simulink model "ES249A_MotAgCorrln"  (R2013b)
settings: Solver=FixedStepDiscrete  SolverMode=SingleTasking  StartTime=0.0  StopTime=1  FixedStep=0.002  RelTol=1e-3
undefined symbols (not defined in the file): FLTINJ_MOTAGCORRLN_MOTAGIDPTSIG, HALFREV_MOTREV_U0P16, MOTAGACORRLNST_CNT_U08, MotAgAMotAgBCorrln, MotAgAMotAgCCorrln, MOTAGBCORRLNST_CNT_U08, MotAgBMotAgCCorrln, MOTAGCCORRLNST_CNT_U08, MOTAGCORRLNERRTHD_MOTREVELEC_U0P16, MOTAGCORRLNNTCFAILSTEP_CNT_U16, MOTAGCORRLNNTCPASSSTEP_CNT_U16, MOTAGMAXSTALLCNTR_CNT_U08, MotAgMeclCorrlnSt, MotAgMeclIdptSig, NtcSts1, sigbuilder_block, SysGlbPrmMotPoleCnt
libraries: simulink x5
(part 3 of 4)

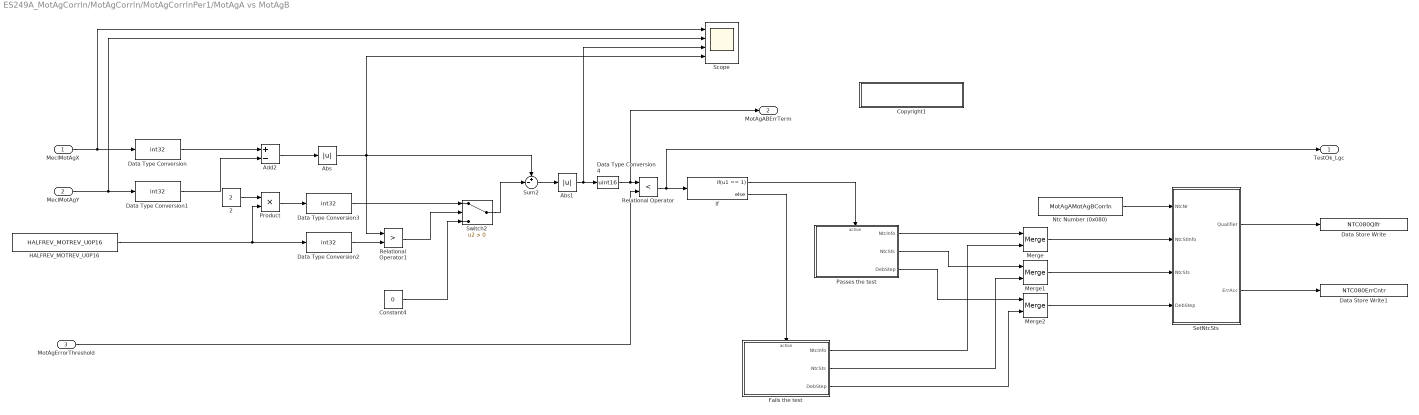
== system ES249A_MotAgCorrln/MotAgCorrln/MotAgCorrlnPer1/MotAgA vs MotAgB ==
  MeclMotAgX : Inport  RequirementInfo={} %GIDa_209a8ec2_f83a_4596_ac14_016e97e43532
  MeclMotAgY : Inport  RequirementInfo={} %GIDa_3879b633_065b_44db_a611_7209c5040c41  Port=2
  MotAgErrorThreshold : Inport  RequirementInfo={} %GIDa_52fd4367_99f4_419f_a569_0cba8f97a327  Port=3
  2 : Constant  Value=2  OutDataTypeStr=int32
  Abs : Abs
  Abs1 : Abs
  Add2 : Sum  Inputs=+-  AccumDataTypeStr=int32
  Constant4 : Constant  Value=0  OutDataTypeStr=int32
  Copyright1 : Subsystem  Description=|  RequirementInfo={} %GIDa_43863c04_fa5e_452c_a1b7_4fa30e8bd61b  mask(Copyright Information){none=on}
      | Copyright info block.                                               
      |                                                                     
      | Place copyright information at the top of every subsystem in design.
      mask prompts: none "No parameters"
      mask help: Place copyright information at the top of every subsystem in design.
      mask Display:
      | NxtrConf = 'Nexteer Confidential';
      | 
      | sys = bdroot; %handle for the current model ("system")
      | first = get_param(sys,'Created');
      | if(isempty(first))
      |     first = datestr(now,'yyyy');
      | else
      |     first = first(end-3:end);  %year is last four digits
      | end
      | 
      | last = get_param(sys,'LastModifiedDate');
      | if isempty(last)
      |     last = datestr(now,'yyyy');
      | else
      |     last = last(end-3:end);
      | end
      | 
      | if strcmp(first,last)
      |     fprintf('%s\nCopyright  %s Nexteer',NxtrConf,first);
      | else
      |     fprintf('%s\n%s%s-%s Nexteer',NxtrConf,char(169),first,last);
      | end
  Data Store Write : DataStoreWrite  RequirementInfo={} %GIDa_9512697d_c087_4109_9134_0a84db0896e8  DataStoreName=NTC080Qlfr
  Data Store Write1 : DataStoreWrite  RequirementInfo={} %GIDa_09fa0ad2_fadc_4e01_82b6_87880c397f4c  DataStoreName=NTC080ErrCntr
  Data Type Conversion{,1..3} (4 alike) : DataTypeConversion  OutDataTypeStr=int32
  Data Type Conversion4 : DataTypeConversion  OutDataTypeStr=uint16
  Fails the test : Subsystem  RequirementInfo={} %GIDa_32330a11_135a_4d4a_b6a9_5738b4884140  TreatAsAtomicUnit=on
  HALFREV_MOTREV_U0P16 : Constant  Value=HALFREV_MOTREV_U0P16  OutDataTypeStr=int32
  If : If  RequirementInfo={} %GIDa_4a7e1530_6c57_410a_8590_40bd88f14402  IfExpression=u1 == 1
  Merge : Merge  RequirementInfo={} %GIDa_5c5d4849_b0d7_417e_8e37_be493b9884db
  Merge1 : Merge  RequirementInfo={} %GIDa_96dc7a19_089f_4a81_91dd_98b954b09d33
  Merge2 : Merge  RequirementInfo={} %GIDa_445cf7d9_fe34_4f83_8f83_84d725eb67cd
  Ntc Number (0x080) : Constant  RequirementInfo={} %GIDa_17484570_857f_4649_8079_9998f179e352  Value=MotAgAMotAgBCorrln
  Passes the test : Subsystem  RequirementInfo={} %GIDa_2e2aa5eb_d2a7_4382_b0d6_a86d4a99b386  TreatAsAtomicUnit=on
  Product : Product
  Relational Operator : RelationalOperator  RequirementInfo={} %GIDa_e81e555f_20f9_4e1d_8333_9ac819d3840d  Operator=<  OutDataTypeStr=boolean
  Relational Operator1 : RelationalOperator  Operator=>  OutDataTypeStr=boolean
  Scope : Scope  NumInputPorts=4
      settings: TimeRange=1  YMin=0~-5~-5~-5  YMax=8~5~5~5
  SetNtcSts : Subsystem  RequirementInfo={} %GIDa_372e5e5c_ac16_4961_ac82_62e12ce3987b  TreatAsAtomicUnit=on
      settings: RTWSystemCode=Inline
  Sum2 : Sum  Inputs=+-|
  Switch2 : Switch  Criteria=u2 > Threshold
  TestOk_Lgc : Outport  RequirementInfo={} %GIDa_58faf550_67b9_443b_9b7a_437f5011a6c4
  MotAgABErrTerm : Outport  RequirementInfo={'linktype_rmi_doors' '0000c47a (/E-STEER Core/SubSystem Specifications/Electrical Actuator/Control Module/FDD Module Requirements/EA4/ES249A_MotAgCorrln)' '#ES249A_116' 'true' 'REQ: ES249A_116' '' } %GIDa_f792b4e5_8164_43e5_9c8c_3a51a3d2addb  Port=2
  wires:
  Relational Operator/1 -> If/1, TestOk_Lgc/1
  If/1 -> Passes the test/Action
  If/2 -> Fails the test/Action
  Ntc Number (0x080)/1 -> SetNtcSts/1(NtcNr)
  Merge/1 -> SetNtcSts/2(NtcStInfo)
  Merge1/1 -> SetNtcSts/3(NtcSts)
  Merge2/1 -> SetNtcSts/4(DebStep)
  Passes the test/1(NtcInfo) -> Merge/1
  Fails the test/1(NtcInfo) -> Merge/2
  Passes the test/2(NtcSts) -> Merge1/1
  Fails the test/2(NtcSts) -> Merge1/2
  Fails the test/3(DebStep) -> Merge2/2
  Passes the test/3(DebStep) -> Merge2/1
  SetNtcSts/1(Qualifier) -> Data Store Write/1
  SetNtcSts/2(ErrAcc) -> Data Store Write1/1
  MotAgErrorThreshold/1 -> Relational Operator/2
  Data Type Conversion/1 -> Add2/1
  Sum2/1 -> Abs1/1
  Data Type Conversion1/1 -> Add2/2
  Switch2/1 -> Sum2/2
  Constant4/1 -> Switch2/3
  Relational Operator1/1 -> Switch2/2
  HALFREV_MOTREV_U0P16/1 -> Product/2, Data Type Conversion2/1
  Abs/1 -> Scope/4, Sum2/1, Relational Operator1/1
  Add2/1 -> Abs/1
  MeclMotAgX/1 -> Scope/1, Data Type Conversion/1
  MeclMotAgY/1 -> Scope/2, Data Type Conversion1/1
  Data Type Conversion2/1 -> Relational Operator1/2
  2/1 -> Product/1
  Product/1 -> Data Type Conversion3/1
  Data Type Conversion3/1 -> Switch2/1
  Abs1/1 -> Data Type Conversion4/1, Scope/3
  Data Type Conversion4/1 -> Relational Operator/1, MotAgABErrTerm/1

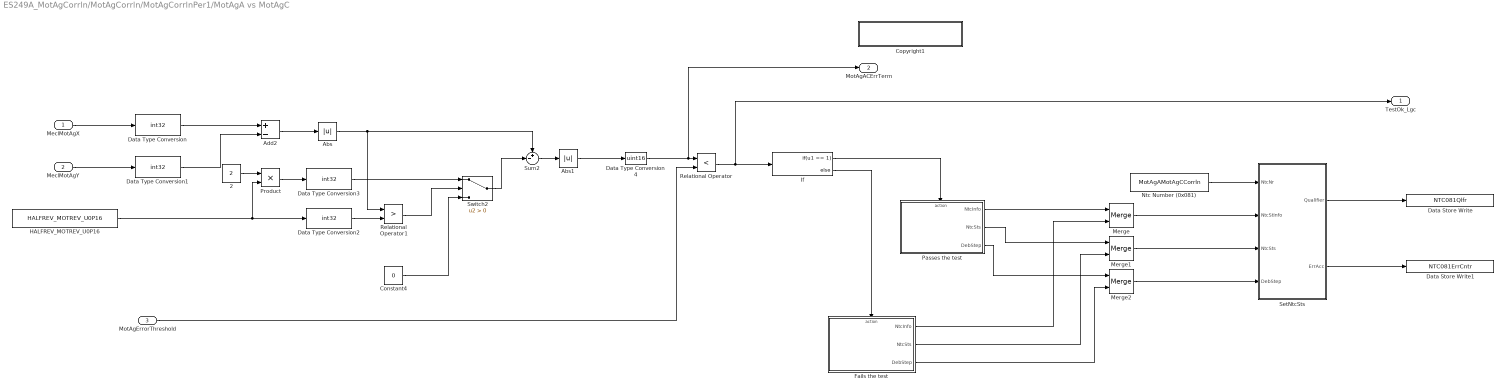
== system ES249A_MotAgCorrln/MotAgCorrln/MotAgCorrlnPer1/MotAgA vs MotAgC ==
  MeclMotAgX : Inport  RequirementInfo={} %GIDa_ca73f5b5_eafe_434b_a911_6609f3f516c8
  MeclMotAgY : Inport  RequirementInfo={} %GIDa_a43669f2_2345_43dd_8255_a23bf60027e6  Port=2
  MotAgErrorThreshold : Inport  RequirementInfo={} %GIDa_293d2f0c_7000_4fd4_9706_6d02dd117e93  Port=3
  2 : Constant  Value=2  OutDataTypeStr=int32
  Abs : Abs
  Abs1 : Abs
  Add2 : Sum  Inputs=+-  AccumDataTypeStr=int32
  Constant4 : Constant  Value=0  OutDataTypeStr=int32
  Copyright1 : Subsystem  Description=|  RequirementInfo={} %GIDa_2297f3bd_4d76_4488_9958_d579b77d02c1  mask(Copyright Information){none=on}
      | Copyright info block.                                               
      |                                                                     
      | Place copyright information at the top of every subsystem in design.
      mask prompts: none "No parameters"
      mask help: Place copyright information at the top of every subsystem in design.
      mask Display:
      | NxtrConf = 'Nexteer Confidential';
      | 
      | sys = bdroot; %handle for the current model ("system")
      | first = get_param(sys,'Created');
      | if(isempty(first))
      |     first = datestr(now,'yyyy');
      | else
      |     first = first(end-3:end);  %year is last four digits
      | end
      | 
      | last = get_param(sys,'LastModifiedDate');
      | if isempty(last)
      |     last = datestr(now,'yyyy');
      | else
      |     last = last(end-3:end);
      | end
      | 
      | if strcmp(first,last)
      |     fprintf('%s\nCopyright  %s Nexteer',NxtrConf,first);
      | else
      |     fprintf('%s\n%s%s-%s Nexteer',NxtrConf,char(169),first,last);
      | end
  Data Store Write : DataStoreWrite  RequirementInfo={} %GIDa_72478395_f981_454c_bb4d_0a88e45525f3  DataStoreName=NTC081Qlfr
  Data Store Write1 : DataStoreWrite  RequirementInfo={} %GIDa_0db287a0_3687_4b20_b932_4d814fe6d91c  DataStoreName=NTC081ErrCntr
  Data Type Conversion{,1..3} (4 alike) : DataTypeConversion  OutDataTypeStr=int32
  Data Type Conversion4 : DataTypeConversion  OutDataTypeStr=uint16
  Fails the test : Subsystem  RequirementInfo={} %GIDa_49fef5d6_5f11_4857_b273_ce522995cb73  TreatAsAtomicUnit=on
  HALFREV_MOTREV_U0P16 : Constant  Value=HALFREV_MOTREV_U0P16  OutDataTypeStr=int32
  If : If  RequirementInfo={} %GIDa_91b41173_b799_4940_951b_3ca3f1c91555  IfExpression=u1 == 1
  Merge : Merge  RequirementInfo={} %GIDa_14c5d993_a2fa_413b_a86d_168b64c7d573
  Merge1 : Merge  RequirementInfo={} %GIDa_c9320e0e_c294_4d17_8556_240a5cb0dfb1
  Merge2 : Merge  RequirementInfo={} %GIDa_945fcc23_377a_4219_9065_ef24679f88cd
  Ntc Number (0x081) : Constant  RequirementInfo={} %GIDa_e90d3b09_c43d_40da_938d_9d742c0ddf76  Value=MotAgAMotAgCCorrln
  Passes the test : Subsystem  RequirementInfo={} %GIDa_e126288c_26d5_4a45_ab77_0ce46127a866  TreatAsAtomicUnit=on
  Product : Product
  Relational Operator : RelationalOperator  RequirementInfo={} %GIDa_6ad4b311_7ce2_4d33_9521_311c03329a1b  Operator=<  OutDataTypeStr=boolean
  Relational Operator1 : RelationalOperator  Operator=>  OutDataTypeStr=boolean
  SetNtcSts : Subsystem  RequirementInfo={} %GIDa_7cf4e5eb_3813_4cd2_9ac5_e73cd08cc7f4  TreatAsAtomicUnit=on
      settings: RTWSystemCode=Inline
  Sum2 : Sum  Inputs=+-|
  Switch2 : Switch  Criteria=u2 > Threshold
  TestOk_Lgc : Outport  RequirementInfo={} %GIDa_0a018449_8aa2_4b67_9646_7371bac07a88
  MotAgACErrTerm : Outport  RequirementInfo={'linktype_rmi_doors' '0000c47a (/E-STEER Core/SubSystem Specifications/Electrical Actuator/Control Module/FDD Module Requirements/EA4/ES249A_MotAgCorrln)' '#ES249A_117' 'true' 'REQ: ES249A_117' '' } %GIDa_a2ba7b60_3fe2_4467_92e3_b3741369c184  Port=2
  wires:
  Relational Operator/1 -> If/1, TestOk_Lgc/1
  If/1 -> Passes the test/Action
  If/2 -> Fails the test/Action
  Ntc Number (0x081)/1 -> SetNtcSts/1(NtcNr)
  Merge/1 -> SetNtcSts/2(NtcStInfo)
  Merge1/1 -> SetNtcSts/3(NtcSts)
  Merge2/1 -> SetNtcSts/4(DebStep)
  Passes the test/1(NtcInfo) -> Merge/1
  Fails the test/1(NtcInfo) -> Merge/2
  Passes the test/2(NtcSts) -> Merge1/1
  Fails the test/2(NtcSts) -> Merge1/2
  Fails the test/3(DebStep) -> Merge2/2
  Passes the test/3(DebStep) -> Merge2/1
  SetNtcSts/1(Qualifier) -> Data Store Write/1
  SetNtcSts/2(ErrAcc) -> Data Store Write1/1
  Abs1/1 -> Data Type Conversion4/1
  MotAgErrorThreshold/1 -> Relational Operator/2
  Data Type Conversion/1 -> Add2/1
  Sum2/1 -> Abs1/1
  Data Type Conversion1/1 -> Add2/2
  Switch2/1 -> Sum2/2
  Constant4/1 -> Switch2/3
  Relational Operator1/1 -> Switch2/2
  HALFREV_MOTREV_U0P16/1 -> Product/2, Data Type Conversion2/1
  Abs/1 -> Sum2/1, Relational Operator1/1
  Add2/1 -> Abs/1
  MeclMotAgX/1 -> Data Type Conversion/1
  MeclMotAgY/1 -> Data Type Conversion1/1
  Data Type Conversion2/1 -> Relational Operator1/2
  2/1 -> Product/1
  Product/1 -> Data Type Conversion3/1
  Data Type Conversion3/1 -> Switch2/1
  Data Type Conversion4/1 -> MotAgACErrTerm/1, Relational Operator/1

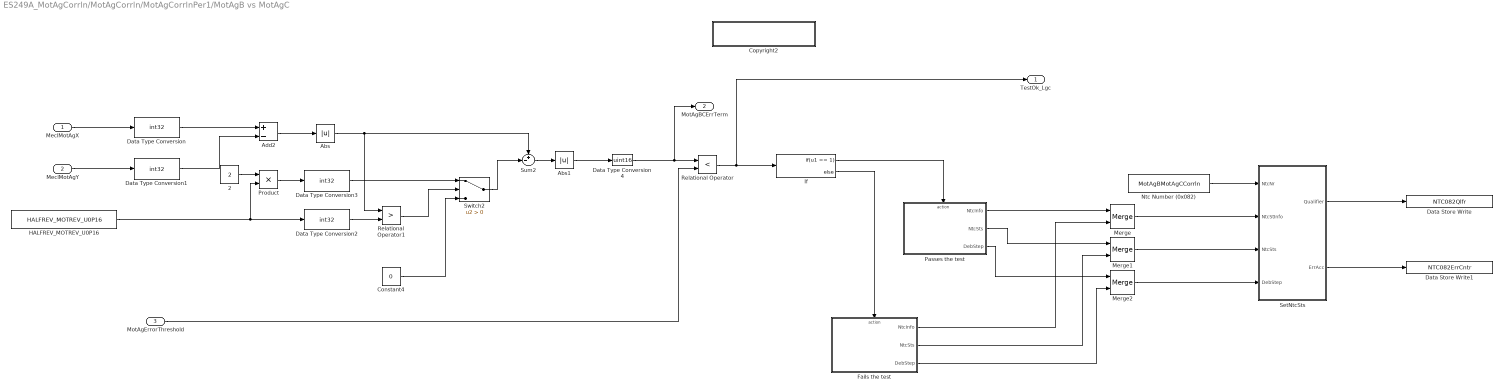
== system ES249A_MotAgCorrln/MotAgCorrln/MotAgCorrlnPer1/MotAgB vs MotAgC ==
  MeclMotAgX : Inport  RequirementInfo={} %GIDa_bf924aab_b5c7_4b3c_951d_c0fbe0c1bb55
  MeclMotAgY : Inport  RequirementInfo={} %GIDa_07ad9c05_b7c9_4d10_b318_38953ab658a8  Port=2
  MotAgErrorThreshold : Inport  RequirementInfo={} %GIDa_2cb4bb85_3f7a_48b7_a9d1_04f72aa7a276  Port=3
  2 : Constant  Value=2  OutDataTypeStr=int32
  Abs : Abs
  Abs1 : Abs
  Add2 : Sum  Inputs=+-  AccumDataTypeStr=int32
  Constant4 : Constant  Value=0  OutDataTypeStr=int32
  Copyright2 : Subsystem  Description=|  RequirementInfo={} %GIDa_151a706e_d981_4739_b788_73043061d7fb  mask(Copyright Information){none=on}
      | Copyright info block.                                               
      |                                                                     
      | Place copyright information at the top of every subsystem in design.
      mask prompts: none "No parameters"
      mask help: Place copyright information at the top of every subsystem in design.
      mask Display:
      | NxtrConf = 'Nexteer Confidential';
      | 
      | sys = bdroot; %handle for the current model ("system")
      | first = get_param(sys,'Created');
      | if(isempty(first))
      |     first = datestr(now,'yyyy');
      | else
      |     first = first(end-3:end);  %year is last four digits
      | end
      | 
      | last = get_param(sys,'LastModifiedDate');
      | if isempty(last)
      |     last = datestr(now,'yyyy');
      | else
      |     last = last(end-3:end);
      | end
      | 
      | if strcmp(first,last)
      |     fprintf('%s\nCopyright  %s Nexteer',NxtrConf,first);
      | else
      |     fprintf('%s\n%s%s-%s Nexteer',NxtrConf,char(169),first,last);
      | end
  Data Store Write : DataStoreWrite  RequirementInfo={} %GIDa_8eb81dab_454a_49f7_9b16_ac976242f325  DataStoreName=NTC082Qlfr
  Data Store Write1 : DataStoreWrite  RequirementInfo={} %GIDa_63ee642a_2bfa_48da_987e_40de90a1b8a9  DataStoreName=NTC082ErrCntr
  Data Type Conversion{,1..3} (4 alike) : DataTypeConversion  OutDataTypeStr=int32
  Data Type Conversion4 : DataTypeConversion  OutDataTypeStr=uint16
  "Fails the test " : Subsystem  RequirementInfo={} %GIDa_f8fb0c70_978f_4e3b_983d_e2d82756bf9b  TreatAsAtomicUnit=on
  HALFREV_MOTREV_U0P16 : Constant  Value=HALFREV_MOTREV_U0P16  OutDataTypeStr=int32
  If : If  RequirementInfo={} %GIDa_d8e22f8c_9e8f_4fa2_b4a1_01dc402be394  IfExpression=u1 == 1
  Merge : Merge  RequirementInfo={} %GIDa_6b0bb93a_8c69_4319_8a50_13213446c0d5
  Merge1 : Merge  RequirementInfo={} %GIDa_af68ae2f_d22d_4760_a231_9874859d41d2
  Merge2 : Merge  RequirementInfo={} %GIDa_e2802f96_b723_4964_a51f_af2ea2fa5b23
  Ntc Number (0x082) : Constant  RequirementInfo={} %GIDa_e1189385_ef24_4fb2_b048_68c7cb7489b1  Value=MotAgBMotAgCCorrln
  Passes the test : Subsystem  RequirementInfo={} %GIDa_82b55705_08f4_4798_b701_46f5356af831  TreatAsAtomicUnit=on
  Product : Product
  Relational Operator : RelationalOperator  RequirementInfo={} %GIDa_38fe0bde_8c6d_4ad7_8dea_b59dbfe668f4  Operator=<  OutDataTypeStr=boolean
  Relational Operator1 : RelationalOperator  Operator=>  OutDataTypeStr=boolean
  SetNtcSts : Subsystem  RequirementInfo={} %GIDa_647bea77_8184_4d0a_9df9_898d529ac2c2  TreatAsAtomicUnit=on
      settings: RTWSystemCode=Inline
  Sum2 : Sum  Inputs=+-|
  Switch2 : Switch  Criteria=u2 > Threshold
  TestOk_Lgc : Outport  RequirementInfo={} %GIDa_45ded846_667e_422a_9bd3_12a64f3f619d
  MotAgBCErrTerm : Outport  RequirementInfo={'linktype_rmi_doors' '0000c47a (/E-STEER Core/SubSystem Specifications/Electrical Actuator/Control Module/FDD Module Requirements/EA4/ES249A_MotAgCorrln)' '#ES249A_118' 'true' 'REQ: ES249A_118' '' } %GIDa_3cdb91e9_0d70_4cbe_a20c_cc0e66a0295d  Port=2
  wires:
  Relational Operator/1 -> If/1, TestOk_Lgc/1
  If/1 -> Passes the test/Action
  If/2 -> "Fails the test "/Action
  Ntc Number (0x082)/1 -> SetNtcSts/1(NtcNr)
  Merge/1 -> SetNtcSts/2(NtcStInfo)
  Merge1/1 -> SetNtcSts/3(NtcSts)
  Merge2/1 -> SetNtcSts/4(DebStep)
  Passes the test/1(NtcInfo) -> Merge/1
  "Fails the test "/1(NtcInfo) -> Merge/2
  Passes the test/2(NtcSts) -> Merge1/1
  "Fails the test "/2(NtcSts) -> Merge1/2
  "Fails the test "/3(DebStep) -> Merge2/2
  Passes the test/3(DebStep) -> Merge2/1
  SetNtcSts/1(Qualifier) -> Data Store Write/1
  SetNtcSts/2(ErrAcc) -> Data Store Write1/1
  Abs1/1 -> Data Type Conversion4/1
  MotAgErrorThreshold/1 -> Relational Operator/2
  Data Type Conversion/1 -> Add2/1
  Sum2/1 -> Abs1/1
  Data Type Conversion1/1 -> Add2/2
  Switch2/1 -> Sum2/2
  Constant4/1 -> Switch2/3
  Relational Operator1/1 -> Switch2/2
  HALFREV_MOTREV_U0P16/1 -> Product/2, Data Type Conversion2/1
  Abs/1 -> Sum2/1, Relational Operator1/1
  Add2/1 -> Abs/1
  MeclMotAgX/1 -> Data Type Conversion/1
  MeclMotAgY/1 -> Data Type Conversion1/1
  Data Type Conversion2/1 -> Relational Operator1/2
  2/1 -> Product/1
  Product/1 -> Data Type Conversion3/1
  Data Type Conversion3/1 -> Switch2/1
  Data Type Conversion4/1 -> MotAgBCErrTerm/1, Relational Operator/1

== system ES249A_MotAgCorrln/MotAgCorrln/MotAgCorrlnPer1/MtrAgA SigAvlCheck ==
  note: Example of PIM declaration for StallCnt State Variable
      |
      | SnsrShoNameSens0StallCntPrev = DataDict.PIM;
      | SnsrShoNameSens0StallCntPrev.LongName = 'SnsrShoNameSens0RollgCntPrev';
      | SnsrShoNameSens0StallCntPrev.Description = 'SnsrShoNameSens0RollgCntPrev';
      | SnsrShoNameSens0StallCntPrev.DocUnits = 'Cnt';
      | SnsrShoNameSens0StallCntPrev.EngDT = dt.u08;
      | SnsrShoNameSens0StallCntPrev.EngInit = 0;
      | SnsrShoNameSens0StallCntPrev.EngMin = 0;
      | SnsrShoNameSens0StallCntPrev.EngMax = 255;
      |
      |
      | *********  Need different state variable for each instance of this  subsystem ********
  note: Example of PIM declaration for RollgCnt State Variable
      |
      | SnsrShoNameSens0RollgCntPrev = DataDict.PIM;
      | SnsrShoNameSens0RollgCntPrev.LongName = 'SnsrShoNameSens0RollgCntPrev';
      | SnsrShoNameSens0RollgCntPrev.Description = 'SnsrShoNameSens0RollgCntPrev';
      | SnsrShoNameSens0RollgCntPrev.DocUnits = 'Cnt';
      | SnsrShoNameSens0RollgCntPrev.EngDT = dt.u08;
      | SnsrShoNameSens0RollgCntPrev.EngInit = 0;
      | SnsrShoNameSens0RollgCntPrev.EngMin = 0;
      | SnsrShoNameSens0RollgCntPrev.EngMax = 255;
      |
      |
      | *********  Need different state variable for each instance of this  subsystem ********
  SigRollgCnt : Inport  OutDataTypeStr=uint8
  SigQlfr : Inport  Port=2  OutDataTypeStr=uint8
  kMaxStallCnt : Inport  Port=3  OutDataTypeStr=uint8
  Copyright1 : Subsystem  Description=|  RequirementInfo={} %GIDa_9c9c1667_19aa_4844_bfe7_7465a4e2bb9e  mask(Copyright Information){none=on}
      | Copyright info block.                                               
      |                                                                     
      | Place copyright information at the top of every subsystem in design.
      mask prompts: none "No parameters"
      mask help: Place copyright information at the top of every subsystem in design.
      mask Display:
      | NxtrConf = 'Nexteer Confidential';
      | 
      | sys = bdroot; %handle for the current model ("system")
      | first = get_param(sys,'Created');
      | if(isempty(first))
      |     first = datestr(now,'yyyy');
      | else
      |     first = first(end-3:end);  %year is last four digits
      | end
      | 
      | last = get_param(sys,'LastModifiedDate');
      | if isempty(last)
      |     last = datestr(now,'yyyy');
      | else
      |     last = last(end-3:end);
      | end
      | 
      | if strcmp(first,last)
      |     fprintf('%s\nCopyright  %s Nexteer',NxtrConf,first);
      | else
      |     fprintf('%s\n%s%s-%s Nexteer',NxtrConf,char(169),first,last);
      | end
  CorrSigAvlChkRev1 : Stateflow chart  TreatAsAtomicUnit=on
  Unit Delay : UnitDelay  SampleTime=-1  StateName=MotAgCorrlnMotAgARollgCntPrev  StateMustResolveToSignalObject=on
      settings: AttributesFormatString=|
      | State Variable:
      | %<StateName>
  Unit Delay1 : UnitDelay  SampleTime=-1  StateName=MotAgCorrlnMotAgAStallCntPrev  StateMustResolveToSignalObject=on
      settings: AttributesFormatString=|
      | State Variable:
      | %<StateName>
  SigAvl : Outport
  wires:
  SigRollgCnt/1 -> Unit Delay/1, CorrSigAvlChkRev1/1(SigRollgCnt)  "SigRollgCnt"
  SigQlfr/1 -> CorrSigAvlChkRev1/2(SigQlfr)  "SigQlfr"
  kMaxStallCnt/1 -> CorrSigAvlChkRev1/3(kMaxStallCnt)  "kMaxStallCnt"
  Unit Delay/1 -> CorrSigAvlChkRev1/4(LstRollgCnt)
  CorrSigAvlChkRev1/2(StallCntOutp) -> Unit Delay1/1
  Unit Delay1/1 -> CorrSigAvlChkRev1/5(LstStallCnt)
  CorrSigAvlChkRev1/1(SigAvl) -> SigAvl/1

== system ES249A_MotAgCorrln/MotAgCorrln/MotAgCorrlnPer1/MtrAgB SigAvlCheck ==
  note: Example of PIM declaration for StallCnt State Variable
      |
      | SnsrShoNameSens0StallCntPrev = DataDict.PIM;
      | SnsrShoNameSens0StallCntPrev.LongName = 'SnsrShoNameSens0RollgCntPrev';
      | SnsrShoNameSens0StallCntPrev.Description = 'SnsrShoNameSens0RollgCntPrev';
      | SnsrShoNameSens0StallCntPrev.DocUnits = 'Cnt';
      | SnsrShoNameSens0StallCntPrev.EngDT = dt.u08;
      | SnsrShoNameSens0StallCntPrev.EngInit = 0;
      | SnsrShoNameSens0StallCntPrev.EngMin = 0;
      | SnsrShoNameSens0StallCntPrev.EngMax = 255;
      |
      |
      | *********  Need different state variable for each instance of this  subsystem ********
  note: Example of PIM declaration for RollgCnt State Variable
      |
      | SnsrShoNameSens0RollgCntPrev = DataDict.PIM;
      | SnsrShoNameSens0RollgCntPrev.LongName = 'SnsrShoNameSens0RollgCntPrev';
      | SnsrShoNameSens0RollgCntPrev.Description = 'SnsrShoNameSens0RollgCntPrev';
      | SnsrShoNameSens0RollgCntPrev.DocUnits = 'Cnt';
      | SnsrShoNameSens0RollgCntPrev.EngDT = dt.u08;
      | SnsrShoNameSens0RollgCntPrev.EngInit = 0;
      | SnsrShoNameSens0RollgCntPrev.EngMin = 0;
      | SnsrShoNameSens0RollgCntPrev.EngMax = 255;
      |
      |
      | *********  Need different state variable for each instance of this  subsystem ********
  SigRollgCnt : Inport  OutDataTypeStr=uint8
  SigQlfr : Inport  Port=2  OutDataTypeStr=uint8
  kMaxStallCnt : Inport  Port=3  OutDataTypeStr=uint8
  Copyright1 : Subsystem  Description=|  RequirementInfo={} %GIDa_9de21268_1023_46e5_9fbe_013ff02661ff  mask(Copyright Information){none=on}
      | Copyright info block.                                               
      |                                                                     
      | Place copyright information at the top of every subsystem in design.
      mask prompts: none "No parameters"
      mask help: Place copyright information at the top of every subsystem in design.
      mask Display:
      | NxtrConf = 'Nexteer Confidential';
      | 
      | sys = bdroot; %handle for the current model ("system")
      | first = get_param(sys,'Created');
      | if(isempty(first))
      |     first = datestr(now,'yyyy');
      | else
      |     first = first(end-3:end);  %year is last four digits
      | end
      | 
      | last = get_param(sys,'LastModifiedDate');
      | if isempty(last)
      |     last = datestr(now,'yyyy');
      | else
      |     last = last(end-3:end);
      | end
      | 
      | if strcmp(first,last)
      |     fprintf('%s\nCopyright  %s Nexteer',NxtrConf,first);
      | else
      |     fprintf('%s\n%s%s-%s Nexteer',NxtrConf,char(169),first,last);
      | end
  CorrSigAvlChkRev1 : Stateflow chart  TreatAsAtomicUnit=on
  Unit Delay : UnitDelay  SampleTime=-1  StateName=MotAgCorrlnMotAgBRollgCntPrev  StateMustResolveToSignalObject=on
      settings: AttributesFormatString=|
      | State Variable:
      | %<StateName>
  Unit Delay1 : UnitDelay  SampleTime=-1  StateName=MotAgCorrlnMotAgBStallCntPrev  StateMustResolveToSignalObject=on
      settings: AttributesFormatString=|
      | State Variable:
      | %<StateName>
  SigAvl : Outport
  wires:
  SigRollgCnt/1 -> Unit Delay/1, CorrSigAvlChkRev1/1(SigRollgCnt)  "SigRollgCnt"
  SigQlfr/1 -> CorrSigAvlChkRev1/2(SigQlfr)  "SigQlfr"
  kMaxStallCnt/1 -> CorrSigAvlChkRev1/3(kMaxStallCnt)  "kMaxStallCnt"
  Unit Delay/1 -> CorrSigAvlChkRev1/4(LstRollgCnt)
  CorrSigAvlChkRev1/2(StallCntOutp) -> Unit Delay1/1
  Unit Delay1/1 -> CorrSigAvlChkRev1/5(LstStallCnt)
  CorrSigAvlChkRev1/1(SigAvl) -> SigAvl/1

== system ES249A_MotAgCorrln/MotAgCorrln/MotAgCorrlnPer1/MtrAgC SigAvlCheck ==
  note: Example of PIM declaration for StallCnt State Variable
      |
      | SnsrShoNameSens0StallCntPrev = DataDict.PIM;
      | SnsrShoNameSens0StallCntPrev.LongName = 'SnsrShoNameSens0RollgCntPrev';
      | SnsrShoNameSens0StallCntPrev.Description = 'SnsrShoNameSens0RollgCntPrev';
      | SnsrShoNameSens0StallCntPrev.DocUnits = 'Cnt';
      | SnsrShoNameSens0StallCntPrev.EngDT = dt.u08;
      | SnsrShoNameSens0StallCntPrev.EngInit = 0;
      | SnsrShoNameSens0StallCntPrev.EngMin = 0;
      | SnsrShoNameSens0StallCntPrev.EngMax = 255;
      |
      |
      | *********  Need different state variable for each instance of this  subsystem ********
  note: Example of PIM declaration for RollgCnt State Variable
      |
      | SnsrShoNameSens0RollgCntPrev = DataDict.PIM;
      | SnsrShoNameSens0RollgCntPrev.LongName = 'SnsrShoNameSens0RollgCntPrev';
      | SnsrShoNameSens0RollgCntPrev.Description = 'SnsrShoNameSens0RollgCntPrev';
      | SnsrShoNameSens0RollgCntPrev.DocUnits = 'Cnt';
      | SnsrShoNameSens0RollgCntPrev.EngDT = dt.u08;
      | SnsrShoNameSens0RollgCntPrev.EngInit = 0;
      | SnsrShoNameSens0RollgCntPrev.EngMin = 0;
      | SnsrShoNameSens0RollgCntPrev.EngMax = 255;
      |
      |
      | *********  Need different state variable for each instance of this  subsystem ********
  SigRollgCnt : Inport  OutDataTypeStr=uint8
  SigQlfr : Inport  Port=2  OutDataTypeStr=uint8
  kMaxStallCnt : Inport  Port=3  OutDataTypeStr=uint8
  Copyright1 : Subsystem  Description=|  RequirementInfo={} %GIDa_602ac125_2bfa_4e71_8efa_b749a3f08ce5  mask(Copyright Information){none=on}
      | Copyright info block.                                               
      |                                                                     
      | Place copyright information at the top of every subsystem in design.
      mask prompts: none "No parameters"
      mask help: Place copyright information at the top of every subsystem in design.
      mask Display:
      | NxtrConf = 'Nexteer Confidential';
      | 
      | sys = bdroot; %handle for the current model ("system")
      | first = get_param(sys,'Created');
      | if(isempty(first))
      |     first = datestr(now,'yyyy');
      | else
      |     first = first(end-3:end);  %year is last four digits
      | end
      | 
      | last = get_param(sys,'LastModifiedDate');
      | if isempty(last)
      |     last = datestr(now,'yyyy');
      | else
      |     last = last(end-3:end);
      | end
      | 
      | if strcmp(first,last)
      |     fprintf('%s\nCopyright  %s Nexteer',NxtrConf,first);
      | else
      |     fprintf('%s\n%s%s-%s Nexteer',NxtrConf,char(169),first,last);
      | end
  CorrSigAvlChkRev1 : Stateflow chart  TreatAsAtomicUnit=on
  Unit Delay : UnitDelay  SampleTime=-1  StateName=MotAgCorrlnMotAgCRollgCntPrev  StateMustResolveToSignalObject=on
      settings: AttributesFormatString=|
      | State Variable:
      | %<StateName>
  Unit Delay1 : UnitDelay  SampleTime=-1  StateName=MotAgCorrlnMotAgCStallCntPrev  StateMustResolveToSignalObject=on
      settings: AttributesFormatString=|
      | State Variable:
      | %<StateName>
  SigAvl : Outport
  wires:
  SigRollgCnt/1 -> Unit Delay/1, CorrSigAvlChkRev1/1(SigRollgCnt)  "SigRollgCnt"
  SigQlfr/1 -> CorrSigAvlChkRev1/2(SigQlfr)  "SigQlfr"
  kMaxStallCnt/1 -> CorrSigAvlChkRev1/3(kMaxStallCnt)  "kMaxStallCnt"
  Unit Delay/1 -> CorrSigAvlChkRev1/4(LstRollgCnt)
  CorrSigAvlChkRev1/2(StallCntOutp) -> Unit Delay1/1
  Unit Delay1/1 -> CorrSigAvlChkRev1/5(LstStallCnt)
  CorrSigAvlChkRev1/1(SigAvl) -> SigAvl/1

== system ES249A_MotAgCorrln/MotAgCorrln/MotAgCorrlnPer1/Pass Action  ==
  MotAgMeclIdptSig1 : Inport
  Action Port : ActionPort  ActionType=then
  Copyright1 : Subsystem  Description=|  mask(Copyright Information){none=on}
      | Copyright info block.                                               
      |                                                                     
      | Place copyright information at the top of every subsystem in design.
      mask prompts: none "No parameters"
      mask help: Place copyright information at the top of every subsystem in design.
      mask Display:
      | NxtrConf = 'Nexteer Confidential';
      | 
      | sys = bdroot; %handle for the current model ("system")
      | first = get_param(sys,'Created');
      | if(isempty(first))
      |     first = datestr(now,'yyyy');
      | else
      |     first = first(end-3:end);  %year is last four digits
      | end
      | 
      | last = get_param(sys,'LastModifiedDate');
      | if isempty(last)
      |     last = datestr(now,'yyyy');
      | else
      |     last = last(end-3:end);
      | end
      | 
      | if strcmp(first,last)
      |     fprintf('%s\nCopyright  %s Nexteer',NxtrConf,first);
      | else
      |     fprintf('%s\n%s%s-%s Nexteer',NxtrConf,char(169),first,last);
      | end
  MotAgMeclIdptSig : Outport
  wires:
  MotAgMeclIdptSig1/1 -> MotAgMeclIdptSig/1

== system ES249A_MotAgCorrln/MotAgCorrln/MotAgCorrlnInit1/Compute Error Threshold/Copyright1 ==

== system ES249A_MotAgCorrln/MotAgCorrln/MotAgCorrlnPer1/Build Correlation Status/Copyright1 ==

== system ES249A_MotAgCorrln/MotAgCorrln/MotAgCorrlnPer1/Fail Action /Copyright1 ==

== system ES249A_MotAgCorrln/MotAgCorrln/MotAgCorrlnPer1/FltInj_u08 /Copyright1 ==

== system ES249A_MotAgCorrln/MotAgCorrln/MotAgCorrlnPer1/GetNtcQlfrSts 0x080 /CopyRight2 ==

== system ES249A_MotAgCorrln/MotAgCorrln/MotAgCorrlnPer1/GetNtcQlfrSts 0x081/CopyRight2 ==

== system ES249A_MotAgCorrln/MotAgCorrln/MotAgCorrlnPer1/GetNtcQlfrSts 0x082/CopyRight2 ==

== system ES249A_MotAgCorrln/MotAgCorrln/MotAgCorrlnPer1/MotAgA vs MotAgB/Copyright1 ==

== system ES249A_MotAgCorrln/MotAgCorrln/MotAgCorrlnPer1/MotAgA vs MotAgB/Fails the test ==
  Action Port : ActionPort  ActionType=else
  Copyright1 : Subsystem  Description=|  mask(Copyright Information){none=on}
      | Copyright info block.                                               
      |                                                                     
      | Place copyright information at the top of every subsystem in design.
      mask prompts: none "No parameters"
      mask help: Place copyright information at the top of every subsystem in design.
      mask Display:
      | NxtrConf = 'Nexteer Confidential';
      | 
      | sys = bdroot; %handle for the current model ("system")
      | first = get_param(sys,'Created');
      | if(isempty(first))
      |     first = datestr(now,'yyyy');
      | else
      |     first = first(end-3:end);  %year is last four digits
      | end
      | 
      | last = get_param(sys,'LastModifiedDate');
      | if isempty(last)
      |     last = datestr(now,'yyyy');
      | else
      |     last = last(end-3:end);
      | end
      | 
      | if strcmp(first,last)
      |     fprintf('%s\nCopyright  %s Nexteer',NxtrConf,first);
      | else
      |     fprintf('%s\n%s%s-%s Nexteer',NxtrConf,char(169),first,last);
      | end
  MOTAGCORRLNNTCFAILSTEP_CNT_U16 : Constant  Value=MOTAGCORRLNNTCFAILSTEP_CNT_U16
  Parameter Byte : Constant  OutDataTypeStr=uint8
  Status Type : Constant  Value=NtcSts1.NTCSTS_PREFAILD
  NtcInfo : Outport  InitialOutput=1
  NtcSts : Outport  Port=2  InitialOutput=NtcSts1.NTCSTS_PREFAILD
  DebStep : Outport  Port=3  InitialOutput=MOTAGCORRLNNTCFAILSTEP_CNT_U16
  wires:
  MOTAGCORRLNNTCFAILSTEP_CNT_U16/1 -> DebStep/1
  Status Type/1 -> NtcSts/1
  Parameter Byte/1 -> NtcInfo/1

== system ES249A_MotAgCorrln/MotAgCorrln/MotAgCorrlnPer1/MotAgA vs MotAgB/Passes the test ==
  Action Port : ActionPort  ActionType=then
  Copyright1 : Subsystem  Description=|  mask(Copyright Information){none=on}
      | Copyright info block.                                               
      |                                                                     
      | Place copyright information at the top of every subsystem in design.
      mask prompts: none "No parameters"
      mask help: Place copyright information at the top of every subsystem in design.
      mask Display:
      | NxtrConf = 'Nexteer Confidential';
      | 
      | sys = bdroot; %handle for the current model ("system")
      | first = get_param(sys,'Created');
      | if(isempty(first))
      |     first = datestr(now,'yyyy');
      | else
      |     first = first(end-3:end);  %year is last four digits
      | end
      | 
      | last = get_param(sys,'LastModifiedDate');
      | if isempty(last)
      |     last = datestr(now,'yyyy');
      | else
      |     last = last(end-3:end);
      | end
      | 
      | if strcmp(first,last)
      |     fprintf('%s\nCopyright  %s Nexteer',NxtrConf,first);
      | else
      |     fprintf('%s\n%s%s-%s Nexteer',NxtrConf,char(169),first,last);
      | end
  MOTAGCORRLNNTCPASSSTEP_CNT_U16 : Constant  Value=MOTAGCORRLNNTCPASSSTEP_CNT_U16
  Parameter Byte Data1 : Constant  Value=0  OutDataTypeStr=uint8
  Status Type : Constant  Value=NtcSts1.NTCSTS_PREPASSD
  NtcInfo : Outport  InitialOutput=0
  NtcSts : Outport  Port=2  InitialOutput=NtcSts1.NTCSTS_PREPASSD
  DebStep : Outport  Port=3  InitialOutput=MOTAGCORRLNNTCPASSSTEP_CNT_U16
  wires:
  MOTAGCORRLNNTCPASSSTEP_CNT_U16/1 -> DebStep/1
  Status Type/1 -> NtcSts/1
  Parameter Byte Data1/1 -> NtcInfo/1

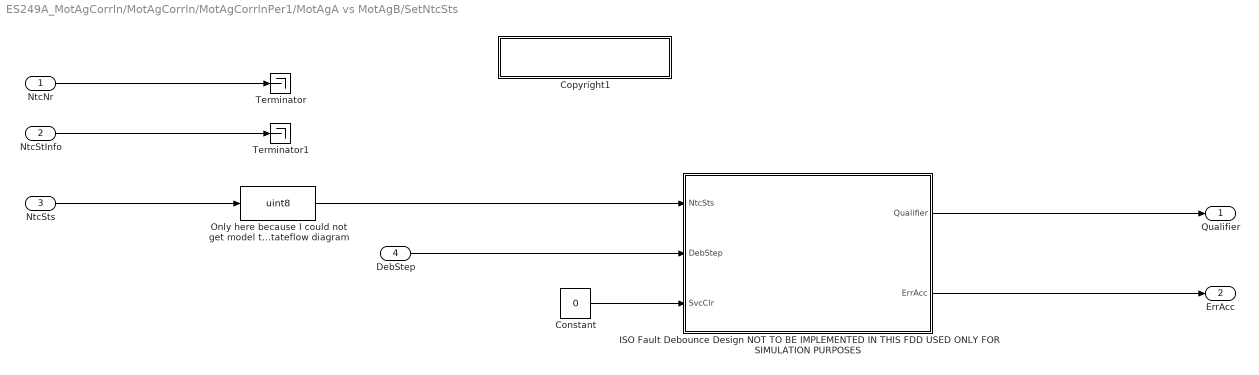
== system ES249A_MotAgCorrln/MotAgCorrln/MotAgCorrlnPer1/MotAgA vs MotAgB/SetNtcSts ==
  NtcNr : Inport
  NtcStInfo : Inport  Port=2
  NtcSts : Inport  Port=3  OutDataTypeStr=Enum: NtcSts1
  DebStep : Inport  Port=4  OutDataTypeStr=uint16
  Constant : Constant  Value=0
  Copyright1 : Subsystem  Description=|  mask(Copyright Information){none=on}
      | Copyright info block.                                               
      |                                                                     
      | Place copyright information at the top of every subsystem in design.
      mask prompts: none "No parameters"
      mask help: Place copyright information at the top of every subsystem in design.
      mask Display:
      | NxtrConf = 'Nexteer Confidential';
      | 
      | sys = bdroot; %handle for the current model ("system")
      | first = get_param(sys,'Created');
      | if(isempty(first))
      |     first = datestr(now,'yyyy');
      | else
      |     first = first(end-3:end);  %year is last four digits
      | end
      | 
      | last = get_param(sys,'LastModifiedDate');
      | if isempty(last)
      |     last = datestr(now,'yyyy');
      | else
      |     last = last(end-3:end);
      | end
      | 
      | if strcmp(first,last)
      |     fprintf('%s\nCopyright  %s Nexteer',NxtrConf,first);
      | else
      |     fprintf('%s\n%s%s-%s Nexteer',NxtrConf,char(169),first,last);
      | end
  ISO Fault Debounce Design NOT TO BE IMPLEMENTED IN THIS FDD USED ONLY FOR SIMULATION PURPOSES : Stateflow chart  TreatAsAtomicUnit=on
  Only here because I could not get model to run with enumerations in the stateflow diagram : DataTypeConversion  OutDataTypeStr=uint8
  Terminator : Terminator
  Terminator1 : Terminator
  Qualifier : Outport
  ErrAcc : Outport  Port=2
  wires:
  Only here because I could not get model to run with enumerations in the stateflow diagram/1 -> ISO Fault Debounce Design NOT TO BE IMPLEMENTED IN THIS FDD USED ONLY FOR SIMULATION PURPOSES/1(NtcSts)
  ISO Fault Debounce Design NOT TO BE IMPLEMENTED IN THIS FDD USED ONLY FOR SIMULATION PURPOSES/2(ErrAcc) -> ErrAcc/1
  Constant/1 -> ISO Fault Debounce Design NOT TO BE IMPLEMENTED IN THIS FDD USED ONLY FOR SIMULATION PURPOSES/3(SvcClr)
  ISO Fault Debounce Design NOT TO BE IMPLEMENTED IN THIS FDD USED ONLY FOR SIMULATION PURPOSES/1(Qualifier) -> Qualifier/1
  DebStep/1 -> ISO Fault Debounce Design NOT TO BE IMPLEMENTED IN THIS FDD USED ONLY FOR SIMULATION PURPOSES/2(DebStep)
  NtcSts/1 -> Only here because I could not get model to run with enumerations in the stateflow diagram/1
  NtcNr/1 -> Terminator/1
  NtcStInfo/1 -> Terminator1/1

== system ES249A_MotAgCorrln/MotAgCorrln/MotAgCorrlnPer1/MotAgA vs MotAgC/Copyright1 ==

== system ES249A_MotAgCorrln/MotAgCorrln/MotAgCorrlnPer1/MotAgA vs MotAgC/Fails the test ==
  Action Port : ActionPort  ActionType=else
  Copyright1 : Subsystem  Description=|  mask(Copyright Information){none=on}
      | Copyright info block.                                               
      |                                                                     
      | Place copyright information at the top of every subsystem in design.
      mask prompts: none "No parameters"
      mask help: Place copyright information at the top of every subsystem in design.
      mask Display:
      | NxtrConf = 'Nexteer Confidential';
      | 
      | sys = bdroot; %handle for the current model ("system")
      | first = get_param(sys,'Created');
      | if(isempty(first))
      |     first = datestr(now,'yyyy');
      | else
      |     first = first(end-3:end);  %year is last four digits
      | end
      | 
      | last = get_param(sys,'LastModifiedDate');
      | if isempty(last)
      |     last = datestr(now,'yyyy');
      | else
      |     last = last(end-3:end);
      | end
      | 
      | if strcmp(first,last)
      |     fprintf('%s\nCopyright  %s Nexteer',NxtrConf,first);
      | else
      |     fprintf('%s\n%s%s-%s Nexteer',NxtrConf,char(169),first,last);
      | end
  MOTAGCORRLNNTCFAILSTEP_CNT_U16 : Constant  Value=MOTAGCORRLNNTCFAILSTEP_CNT_U16
  Parameter Byte : Constant  OutDataTypeStr=uint8
  Status Type : Constant  Value=NtcSts1.NTCSTS_PREFAILD
  NtcInfo : Outport  InitialOutput=1
  NtcSts : Outport  Port=2  InitialOutput=NtcSts1.NTCSTS_PREFAILD
  DebStep : Outport  Port=3  InitialOutput=MOTAGCORRLNNTCFAILSTEP_CNT_U16
  wires:
  MOTAGCORRLNNTCFAILSTEP_CNT_U16/1 -> DebStep/1
  Status Type/1 -> NtcSts/1
  Parameter Byte/1 -> NtcInfo/1

== system ES249A_MotAgCorrln/MotAgCorrln/MotAgCorrlnPer1/MotAgA vs MotAgC/Passes the test ==
  Action Port : ActionPort  ActionType=then
  Copyright1 : Subsystem  Description=|  mask(Copyright Information){none=on}
      | Copyright info block.                                               
      |                                                                     
      | Place copyright information at the top of every subsystem in design.
      mask prompts: none "No parameters"
      mask help: Place copyright information at the top of every subsystem in design.
      mask Display:
      | NxtrConf = 'Nexteer Confidential';
      | 
      | sys = bdroot; %handle for the current model ("system")
      | first = get_param(sys,'Created');
      | if(isempty(first))
      |     first = datestr(now,'yyyy');
      | else
      |     first = first(end-3:end);  %year is last four digits
      | end
      | 
      | last = get_param(sys,'LastModifiedDate');
      | if isempty(last)
      |     last = datestr(now,'yyyy');
      | else
      |     last = last(end-3:end);
      | end
      | 
      | if strcmp(first,last)
      |     fprintf('%s\nCopyright  %s Nexteer',NxtrConf,first);
      | else
      |     fprintf('%s\n%s%s-%s Nexteer',NxtrConf,char(169),first,last);
      | end
  MOTAGCORRLNNTCPASSSTEP_CNT_U16 : Constant  Value=MOTAGCORRLNNTCPASSSTEP_CNT_U16
  Parameter Byte Data1 : Constant  Value=0  OutDataTypeStr=uint8
  Status Type : Constant  Value=NtcSts1.NTCSTS_PREPASSD
  NtcInfo : Outport  InitialOutput=0
  NtcSts : Outport  Port=2  InitialOutput=NtcSts1.NTCSTS_PREPASSD
  DebStep : Outport  Port=3  InitialOutput=MOTAGCORRLNNTCPASSSTEP_CNT_U16
  wires:
  MOTAGCORRLNNTCPASSSTEP_CNT_U16/1 -> DebStep/1
  Status Type/1 -> NtcSts/1
  Parameter Byte Data1/1 -> NtcInfo/1

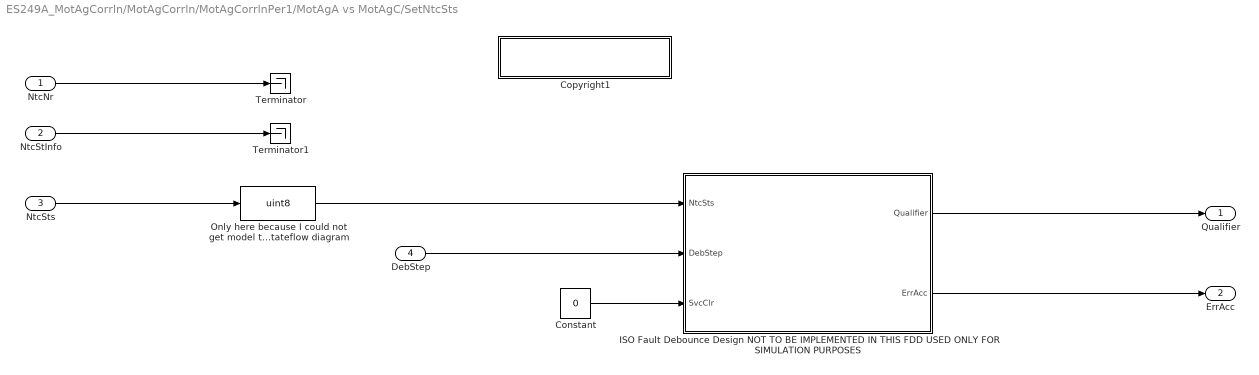
== system ES249A_MotAgCorrln/MotAgCorrln/MotAgCorrlnPer1/MotAgA vs MotAgC/SetNtcSts ==
  NtcNr : Inport
  NtcStInfo : Inport  Port=2
  NtcSts : Inport  Port=3  OutDataTypeStr=Enum: NtcSts1
  DebStep : Inport  Port=4
  Constant : Constant  Value=0
  Copyright1 : Subsystem  Description=|  mask(Copyright Information){none=on}
      | Copyright info block.                                               
      |                                                                     
      | Place copyright information at the top of every subsystem in design.
      mask prompts: none "No parameters"
      mask help: Place copyright information at the top of every subsystem in design.
      mask Display:
      | NxtrConf = 'Nexteer Confidential';
      | 
      | sys = bdroot; %handle for the current model ("system")
      | first = get_param(sys,'Created');
      | if(isempty(first))
      |     first = datestr(now,'yyyy');
      | else
      |     first = first(end-3:end);  %year is last four digits
      | end
      | 
      | last = get_param(sys,'LastModifiedDate');
      | if isempty(last)
      |     last = datestr(now,'yyyy');
      | else
      |     last = last(end-3:end);
      | end
      | 
      | if strcmp(first,last)
      |     fprintf('%s\nCopyright  %s Nexteer',NxtrConf,first);
      | else
      |     fprintf('%s\n%s%s-%s Nexteer',NxtrConf,char(169),first,last);
      | end
  ISO Fault Debounce Design NOT TO BE IMPLEMENTED IN THIS FDD USED ONLY FOR SIMULATION PURPOSES : Stateflow chart  TreatAsAtomicUnit=on
  Only here because I could not get model to run with enumerations in the stateflow diagram : DataTypeConversion  OutDataTypeStr=uint8
  Terminator : Terminator
  Terminator1 : Terminator
  Qualifier : Outport
  ErrAcc : Outport  Port=2
  wires:
  Only here because I could not get model to run with enumerations in the stateflow diagram/1 -> ISO Fault Debounce Design NOT TO BE IMPLEMENTED IN THIS FDD USED ONLY FOR SIMULATION PURPOSES/1(NtcSts)
  ISO Fault Debounce Design NOT TO BE IMPLEMENTED IN THIS FDD USED ONLY FOR SIMULATION PURPOSES/2(ErrAcc) -> ErrAcc/1
  Constant/1 -> ISO Fault Debounce Design NOT TO BE IMPLEMENTED IN THIS FDD USED ONLY FOR SIMULATION PURPOSES/3(SvcClr)
  ISO Fault Debounce Design NOT TO BE IMPLEMENTED IN THIS FDD USED ONLY FOR SIMULATION PURPOSES/1(Qualifier) -> Qualifier/1
  DebStep/1 -> ISO Fault Debounce Design NOT TO BE IMPLEMENTED IN THIS FDD USED ONLY FOR SIMULATION PURPOSES/2(DebStep)
  NtcSts/1 -> Only here because I could not get model to run with enumerations in the stateflow diagram/1
  NtcNr/1 -> Terminator/1
  NtcStInfo/1 -> Terminator1/1

== system ES249A_MotAgCorrln/MotAgCorrln/MotAgCorrlnPer1/MotAgB vs MotAgC/Copyright2 ==

== system ES249A_MotAgCorrln/MotAgCorrln/MotAgCorrlnPer1/MotAgB vs MotAgC/Fails the test  ==
  Action Port : ActionPort  ActionType=else
  Copyright1 : Subsystem  Description=|  mask(Copyright Information){none=on}
      | Copyright info block.                                               
      |                                                                     
      | Place copyright information at the top of every subsystem in design.
      mask prompts: none "No parameters"
      mask help: Place copyright information at the top of every subsystem in design.
      mask Display:
      | NxtrConf = 'Nexteer Confidential';
      | 
      | sys = bdroot; %handle for the current model ("system")
      | first = get_param(sys,'Created');
      | if(isempty(first))
      |     first = datestr(now,'yyyy');
      | else
      |     first = first(end-3:end);  %year is last four digits
      | end
      | 
      | last = get_param(sys,'LastModifiedDate');
      | if isempty(last)
      |     last = datestr(now,'yyyy');
      | else
      |     last = last(end-3:end);
      | end
      | 
      | if strcmp(first,last)
      |     fprintf('%s\nCopyright  %s Nexteer',NxtrConf,first);
      | else
      |     fprintf('%s\n%s%s-%s Nexteer',NxtrConf,char(169),first,last);
      | end
  MOTAGCORRLNNTCPASSSTEP_CNT_U16 : Constant  Value=MOTAGCORRLNNTCFAILSTEP_CNT_U16
  Parameter Byte : Constant  OutDataTypeStr=uint8
  Status Type : Constant  Value=NtcSts1.NTCSTS_PREFAILD
  NtcInfo : Outport  InitialOutput=1
  NtcSts : Outport  Port=2  InitialOutput=NtcSts1.NTCSTS_PREFAILD
  DebStep : Outport  Port=3  InitialOutput=MOTAGCORRLNNTCFAILSTEP_CNT_U16
  wires:
  MOTAGCORRLNNTCPASSSTEP_CNT_U16/1 -> DebStep/1
  Status Type/1 -> NtcSts/1
  Parameter Byte/1 -> NtcInfo/1

== system ES249A_MotAgCorrln/MotAgCorrln/MotAgCorrlnPer1/MotAgB vs MotAgC/Passes the test ==
  Action Port : ActionPort  ActionType=then
  Copyright1 : Subsystem  Description=|  mask(Copyright Information){none=on}
      | Copyright info block.                                               
      |                                                                     
      | Place copyright information at the top of every subsystem in design.
      mask prompts: none "No parameters"
      mask help: Place copyright information at the top of every subsystem in design.
      mask Display:
      | NxtrConf = 'Nexteer Confidential';
      | 
      | sys = bdroot; %handle for the current model ("system")
      | first = get_param(sys,'Created');
      | if(isempty(first))
      |     first = datestr(now,'yyyy');
      | else
      |     first = first(end-3:end);  %year is last four digits
      | end
      | 
      | last = get_param(sys,'LastModifiedDate');
      | if isempty(last)
      |     last = datestr(now,'yyyy');
      | else
      |     last = last(end-3:end);
      | end
      | 
      | if strcmp(first,last)
      |     fprintf('%s\nCopyright  %s Nexteer',NxtrConf,first);
      | else
      |     fprintf('%s\n%s%s-%s Nexteer',NxtrConf,char(169),first,last);
      | end
  MOTAGCORRLNNTCPASSSTEP_CNT_U16 : Constant  Value=MOTAGCORRLNNTCPASSSTEP_CNT_U16
  Parameter Byte Data1 : Constant  Value=0  OutDataTypeStr=uint8
  Status Type : Constant  Value=NtcSts1.NTCSTS_PREPASSD
  NtcInfo : Outport  InitialOutput=0
  NtcSts : Outport  Port=2  InitialOutput=NtcSts1.NTCSTS_PREPASSD
  DebStep : Outport  Port=3  InitialOutput=MOTAGCORRLNNTCPASSSTEP_CNT_U16
  wires:
  MOTAGCORRLNNTCPASSSTEP_CNT_U16/1 -> DebStep/1
  Status Type/1 -> NtcSts/1
  Parameter Byte Data1/1 -> NtcInfo/1

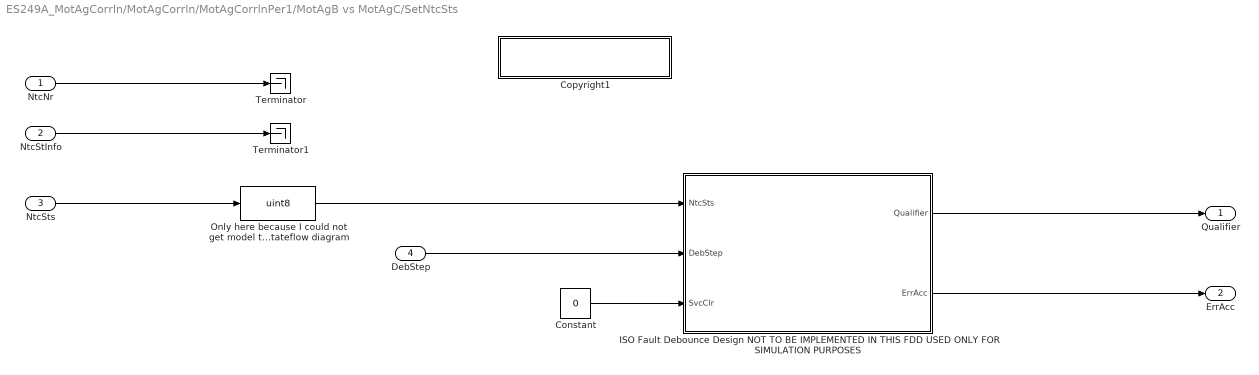
== system ES249A_MotAgCorrln/MotAgCorrln/MotAgCorrlnPer1/MotAgB vs MotAgC/SetNtcSts ==
  NtcNr : Inport
  NtcStInfo : Inport  Port=2
  NtcSts : Inport  Port=3  OutDataTypeStr=Enum: NtcSts1
  DebStep : Inport  Port=4
  Constant : Constant  Value=0
  Copyright1 : Subsystem  Description=|  mask(Copyright Information){none=on}
      | Copyright info block.                                               
      |                                                                     
      | Place copyright information at the top of every subsystem in design.
      mask prompts: none "No parameters"
      mask help: Place copyright information at the top of every subsystem in design.
      mask Display:
      | NxtrConf = 'Nexteer Confidential';
      | 
      | sys = bdroot; %handle for the current model ("system")
      | first = get_param(sys,'Created');
      | if(isempty(first))
      |     first = datestr(now,'yyyy');
      | else
      |     first = first(end-3:end);  %year is last four digits
      | end
      | 
      | last = get_param(sys,'LastModifiedDate');
      | if isempty(last)
      |     last = datestr(now,'yyyy');
      | else
      |     last = last(end-3:end);
      | end
      | 
      | if strcmp(first,last)
      |     fprintf('%s\nCopyright  %s Nexteer',NxtrConf,first);
      | else
      |     fprintf('%s\n%s%s-%s Nexteer',NxtrConf,char(169),first,last);
      | end
  ISO Fault Debounce Design NOT TO BE IMPLEMENTED IN THIS FDD USED ONLY FOR SIMULATION PURPOSES : Stateflow chart  TreatAsAtomicUnit=on
  Only here because I could not get model to run with enumerations in the stateflow diagram : DataTypeConversion  OutDataTypeStr=uint8
  Terminator : Terminator
  Terminator1 : Terminator
  Qualifier : Outport
  ErrAcc : Outport  Port=2
  wires:
  Only here because I could not get model to run with enumerations in the stateflow diagram/1 -> ISO Fault Debounce Design NOT TO BE IMPLEMENTED IN THIS FDD USED ONLY FOR SIMULATION PURPOSES/1(NtcSts)
  ISO Fault Debounce Design NOT TO BE IMPLEMENTED IN THIS FDD USED ONLY FOR SIMULATION PURPOSES/2(ErrAcc) -> ErrAcc/1
  Constant/1 -> ISO Fault Debounce Design NOT TO BE IMPLEMENTED IN THIS FDD USED ONLY FOR SIMULATION PURPOSES/3(SvcClr)
  ISO Fault Debounce Design NOT TO BE IMPLEMENTED IN THIS FDD USED ONLY FOR SIMULATION PURPOSES/1(Qualifier) -> Qualifier/1
  DebStep/1 -> ISO Fault Debounce Design NOT TO BE IMPLEMENTED IN THIS FDD USED ONLY FOR SIMULATION PURPOSES/2(DebStep)
  NtcSts/1 -> Only here because I could not get model to run with enumerations in the stateflow diagram/1
  NtcNr/1 -> Terminator/1
  NtcStInfo/1 -> Terminator1/1

== system ES249A_MotAgCorrln/MotAgCorrln/MotAgCorrlnPer1/MtrAgA SigAvlCheck/Copyright1 ==

== system ES249A_MotAgCorrln/MotAgCorrln/MotAgCorrlnPer1/MtrAgB SigAvlCheck/Copyright1 ==

== system ES249A_MotAgCorrln/MotAgCorrln/MotAgCorrlnPer1/MtrAgC SigAvlCheck/Copyright1 ==

== system ES249A_MotAgCorrln/MotAgCorrln/MotAgCorrlnPer1/Pass Action /Copyright1 ==

== system ES249A_MotAgCorrln/MotAgCorrln/MotAgCorrlnPer1/MotAgA vs MotAgB/Fails the test/Copyright1 ==

== system ES249A_MotAgCorrln/MotAgCorrln/MotAgCorrlnPer1/MotAgA vs MotAgB/Passes the test/Copyright1 ==

== system ES249A_MotAgCorrln/MotAgCorrln/MotAgCorrlnPer1/MotAgA vs MotAgB/SetNtcSts/Copyright1 ==

== system ES249A_MotAgCorrln/MotAgCorrln/MotAgCorrlnPer1/MotAgA vs MotAgC/Fails the test/Copyright1 ==

== system ES249A_MotAgCorrln/MotAgCorrln/MotAgCorrlnPer1/MotAgA vs MotAgC/Passes the test/Copyright1 ==

== system ES249A_MotAgCorrln/MotAgCorrln/MotAgCorrlnPer1/MotAgA vs MotAgC/SetNtcSts/Copyright1 ==

== system ES249A_MotAgCorrln/MotAgCorrln/MotAgCorrlnPer1/MotAgB vs MotAgC/Fails the test /Copyright1 ==

== system ES249A_MotAgCorrln/MotAgCorrln/MotAgCorrlnPer1/MotAgB vs MotAgC/Passes the test/Copyright1 ==

== system ES249A_MotAgCorrln/MotAgCorrln/MotAgCorrlnPer1/MotAgB vs MotAgC/SetNtcSts/Copyright1 ==
